simulink model "Plantv5"  (R2017a)
settings: Solver=FixedStepAuto  StartTime=0.0  StopTime=6000  FixedStep=.1  MaxStep=4.0  MinStep=.001  RelTol=1e-6
values from neighbouring files (symbols this model uses):
  B0 = 3.12e-5    (= 3.12e-05)    [starshot_DC_KD_setup.m]    (also in starshot_DC_setup.m; starshotmath.m; temp.m)
  G = 6.67e-11    [starshot_DC_KD_setup.m]    (also in starshot_DC_setup.m; temp.m)
  M_Earth = 5.972e24    (= 5.972e+24)    [starshot_DC_KD_setup.m]    (also in starshot_DC_setup.m; temp.m)
  q0 = [qmatlab(2:4),qmatlab(1)]'    [starshot_DC_KD_setup.m]    (also in starshot_DC_setup.m; temp.m)
  R_Earth = 6.378e6    (= 6378000)    [starshot_DC_KD_setup.m]    (also in starshot_DC_setup.m; temp.m)
undefined symbols (not defined in the file or in its folder): DiscIntNeverNeededParam, starshot
libraries: vrlib x2
settings Model: Creator=armen  LastModifiedBy=armen
settings OptimizationCC: DefaultParameterBehavior=Inlined  UseDivisionForNetSlopeComputation=on  UseFloatMulNetSlope=on  InlineInvariantSignals=on  PassReuseOutputArgsAs=Individual arguments  ZeroExternalMemoryAtStartup=off  ZeroInternalMemoryAtStartup=off  NoFixptDivByZeroProtection=on  EfficientFloat2IntCast=on  LifeSpan=1
settings DebuggingCC: ParameterTunabilityLossMsg=error  FrameProcessingCompatibilityMsg=none
settings HardwareCC: ProdBitPerPointer=32  ProdBitPerSizeT=32  ProdBitPerPtrDiffT=32  ProdLargestAtomicInteger=Long  ProdLargestAtomicFloat=Double  ProdWordSize=32  ProdHWDeviceType=ARM Compatible->ARM Cortex
settings SFSimCC: MATLABDynamicMemAlloc=off
settings RTWCC: SystemTargetFile=ert.tlc  TLCOptions=-aAlwaysIncludeCustomSrc=1  GenCodeOnly=on  TemplateMakefile=ert_default_tmf  Description=Embedded Coder  GenerateReport=on  IncludeHyperlinkInReport=on  LaunchReport=on  TargetLang=C++  GenerateTraceInfo=on  GenerateTraceReport=on  GenerateTraceReportSl=on  GenerateTraceReportSf=on  GenerateTraceReportEml=on
settings CodeAppCC: ForceParamTrailComments=on  IgnoreCustomStorageClasses=off  OperatorAnnotations=on  SimulinkDataObjDesc=on  SFDataObjDesc=on  MATLABFcnDesc=on  CustomSymbolStrGlobalVar=rt$N$M  CustomSymbolStrType=$N$M  CustomSymbolStrFcn=$N$M$F  CustomSymbolStrMacro=$N$M  InsertBlockDesc=on  MATLABSourceComments=on
settings ERTTargetCC: TargetLangStandard=C++03 (ISO)  GenerateSampleERTMain=on  IncludeMdlTerminateFcn=off  CombineSignalStateStructs=on  SupportAbsoluteTime=off  MultiInstanceERTCode=on  CodeInterfacePackaging=C++ class  SupportComplex=off  SupportNonInlinedSFcns=on  InlinedParameterPlacement=NonHierarchical  RootIOFormat=Structure reference  ERTCustomFileTemplate=example_file_process.tlc  ERTFilePackagingFormat=CompactWithDataFile

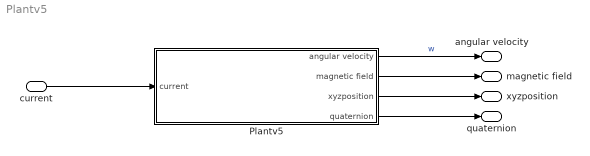
== system Plantv5 ==
  current : Inport  OutDataTypeStr=double  PortDimensions=3  SampleTime=[0.10000000000000001 0]  Interpolate=off
  Plantv5 : Subsystem  Tag=starshotsimv5  TreatAsAtomicUnit=on
      settings: RTWSystemCode=Inline
  angular velocity : Outport  OutDataTypeStr=double  PortDimensions=3  SampleTime=[0.10000000000000001 0]
  magnetic field : Outport  Port=2  OutDataTypeStr=double  PortDimensions=3  SampleTime=[0.10000000000000001 0]
  xyzposition : Outport  Port=3  OutDataTypeStr=double  PortDimensions=3  SampleTime=[0.10000000000000001 0]
  quaternion : Outport  Port=4  OutDataTypeStr=double  PortDimensions=4  SampleTime=[0.10000000000000001 0]
  wires:
  current/1 -> Plantv5/1(current)
  Plantv5/1(angular velocity) -> angular velocity/1  "w"
  Plantv5/2(magnetic field) -> magnetic field/1
  Plantv5/3(xyzposition) -> xyzposition/1
  Plantv5/4(quaternion) -> quaternion/1

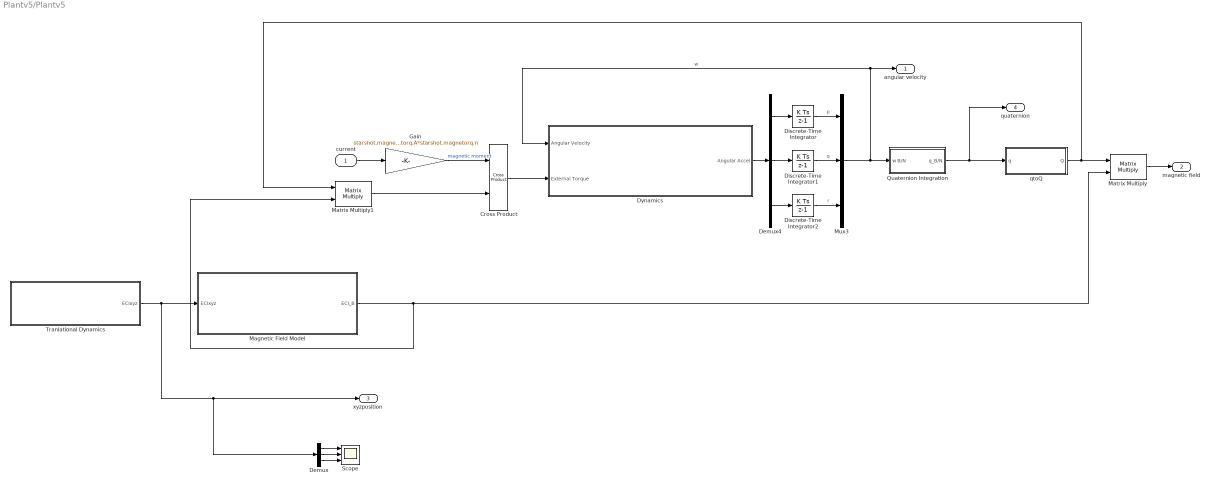
== system Plantv5/Plantv5 ==
  current : Inport
  Cross Product : vrlib/Utilities/Cross Product
      settings: SourceProductBaseCode=VR
  Demux : Demux  Outputs=3
  Demux4 : Demux  Outputs=3
  Discrete-Time Integrator : DiscreteIntegrator  InitialCondition=starshot.IC.w(1)  InitialConditionSetting=State (most efficient)  SampleTime=-1  ICPrevOutput=DiscIntNeverNeededParam  ICPrevScaledInput=DiscIntNeverNeededParam
  Discrete-Time Integrator1 : DiscreteIntegrator  InitialCondition=starshot.IC.w(2)  InitialConditionSetting=State (most efficient)  SampleTime=-1  ICPrevOutput=DiscIntNeverNeededParam  ICPrevScaledInput=DiscIntNeverNeededParam
  Discrete-Time Integrator2 : DiscreteIntegrator  InitialCondition=starshot.IC.w(3)  InitialConditionSetting=State (most efficient)  SampleTime=-1  ICPrevOutput=DiscIntNeverNeededParam  ICPrevScaledInput=DiscIntNeverNeededParam
  Dynamics : Subsystem  TreatAsAtomicUnit=on
  Gain : Gain  Gain=starshot.magnetorq.A*starshot.magnetorq.n
  Magnetic Field Model : Subsystem  TreatAsAtomicUnit=on
  Matrix Multiply : Product  Multiplication=Matrix(*)
  Matrix Multiply1 : Product  Multiplication=Matrix(*)
  Mux3 : Mux  Inputs=3
  Quaternion Integration : Subsystem
  Scope : Scope  NumInputPorts=3
  Tranlational Dynamics : Subsystem  TreatAsAtomicUnit=on
  qtoQ : Subsystem  TreatAsAtomicUnit=on
  angular velocity : Outport
  magnetic field : Outport  Port=2
  xyzposition : Outport  Port=3
  quaternion : Outport  Port=4
  wires:
  Matrix Multiply1/1 -> Cross Product/2
  qtoQ/1(Q) -> Matrix Multiply/1, Matrix Multiply1/1
  Demux/3 -> Scope/3
  Demux/1 -> Scope/1
  Demux/2 -> Scope/2
  Demux4/2 -> Discrete-Time Integrator1/1
  Discrete-Time Integrator/1 -> Mux3/1  "p"
  Cross Product/1 -> Dynamics/2(External Torque)
  Gain/1 -> Cross Product/1  "magnetic moment"
  current/1 -> Gain/1
  Mux3/1 -> angular velocity/1, Dynamics/1(Angular Velocity), Quaternion Integration/1(w B/N)  "w"
  Dynamics/1(Angular Accel) -> Demux4/1
  Quaternion Integration/1(q_B/N) -> qtoQ/1(q), quaternion/1
  Tranlational Dynamics/1(ECIxyz) -> Magnetic Field Model/1(ECIxyz), xyzposition/1, Demux/1
  Demux4/1 -> Discrete-Time Integrator/1
  Demux4/3 -> Discrete-Time Integrator2/1
  Discrete-Time Integrator2/1 -> Mux3/3  "r"
  Discrete-Time Integrator1/1 -> Mux3/2  "q"
  Magnetic Field Model/1(ECI_B) -> Matrix Multiply/2, Matrix Multiply1/2
  Matrix Multiply/1 -> magnetic field/1

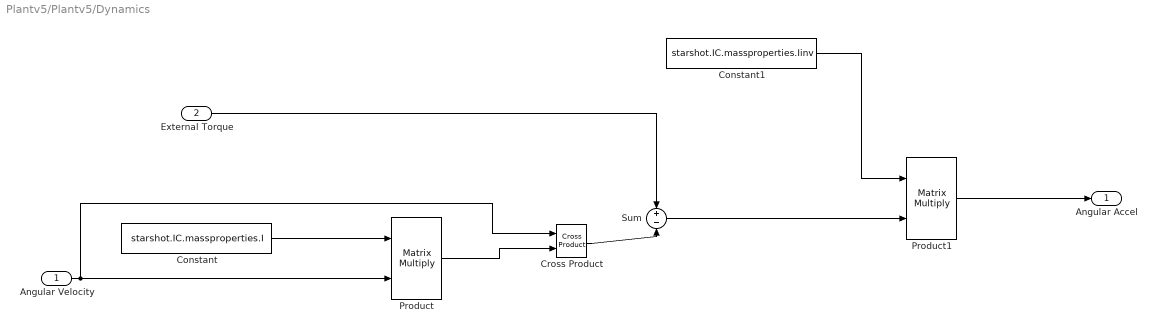
== system Plantv5/Plantv5/Dynamics ==
  Angular Velocity : Inport
  External Torque : Inport  Port=2
  Constant : Constant  Value=starshot.IC.massproperties.I
  Constant1 : Constant  Value=starshot.IC.massproperties.Iinv
  Cross Product : vrlib/Utilities/Cross Product
      settings: SourceProductBaseCode=VR
  Product : Product  Multiplication=Matrix(*)
  Product1 : Product  Multiplication=Matrix(*)
  Sum : Sum  Inputs=+-
  Angular Accel : Outport
  wires:
  Sum/1 -> Product1/2
  Product1/1 -> Angular Accel/1
  Constant1/1 -> Product1/1
  External Torque/1 -> Sum/1
  Product/1 -> Cross Product/2
  Cross Product/1 -> Sum/2
  Constant/1 -> Product/1
  Angular Velocity/1 -> Product/2, Cross Product/1

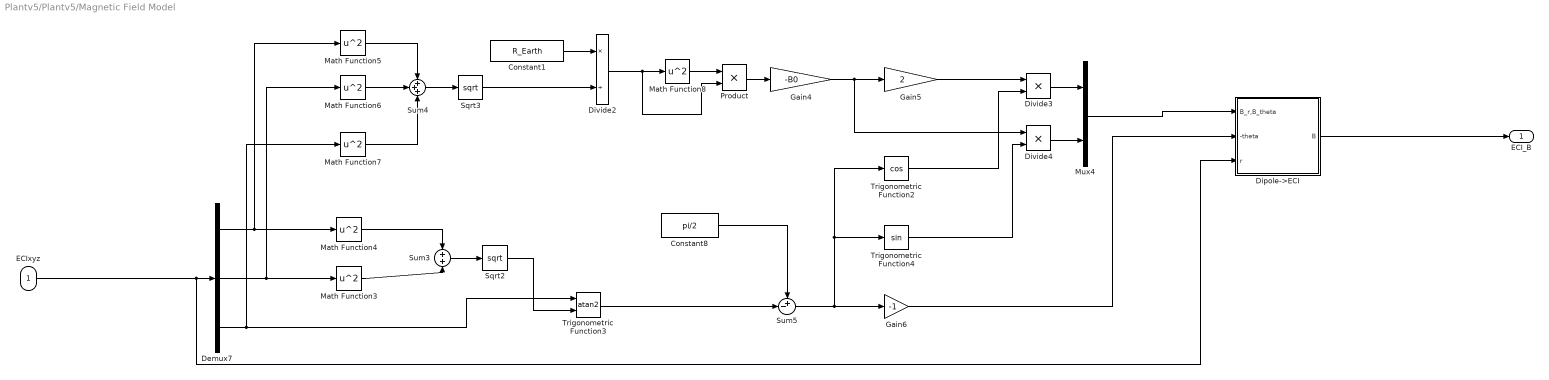
== system Plantv5/Plantv5/Magnetic Field Model ==
  ECIxyz : Inport
  Constant1 : Constant  Value=R_Earth
  Constant8 : Constant  Value=pi/2
  Demux7 : Demux  Outputs=3
  Dipole->ECI : Subsystem  TreatAsAtomicUnit=on
  Divide2 : Product  Inputs=*/
  Divide3 : Product  Inputs=**
  Divide4 : Product  Inputs=**
  Gain4 : Gain  Gain=-B0
  Gain5 : Gain  Gain=2
  Gain6 : Gain  Gain=-1
  Math Function{3..8} (6 alike) : Math  Operator=square  SaturateOnIntegerOverflow=on
  Mux4 : Mux  Inputs=2
  Product : Product
  Sqrt2 : Sqrt  SaturateOnIntegerOverflow=on
  Sqrt3 : Sqrt  SaturateOnIntegerOverflow=on
  Sum3 : Sum
  Sum4 : Sum  Inputs=+++
  Sum5 : Sum  Inputs=+-|
  Trigonometric Function2 : Trigonometry  Operator=cos
  Trigonometric Function3 : Trigonometry  Operator=atan2
  Trigonometric Function4 : Trigonometry
  ECI_B : Outport
  wires:
  ECIxyz/1 -> Demux7/1, Dipole->ECI/3(r)
  Divide3/1 -> Mux4/1
  Dipole->ECI/1(B) -> ECI_B/1
  Mux4/1 -> Dipole->ECI/1(B_r,B_theta)
  Constant8/1 -> Sum5/1
  Trigonometric Function3/1 -> Sum5/2
  Divide4/1 -> Mux4/2
  Gain6/1 -> Dipole->ECI/2(-theta)
  Trigonometric Function4/1 -> Divide4/2
  Sum5/1 -> Gain6/1, Trigonometric Function4/1, Trigonometric Function2/1
  Demux7/2 -> Math Function3/1, Math Function6/1
  Math Function6/1 -> Sum4/2
  Trigonometric Function2/1 -> Divide3/2
  Gain4/1 -> Divide4/1, Gain5/1
  Demux7/1 -> Math Function4/1, Math Function5/1
  Math Function3/1 -> Sum3/2
  Sum3/1 -> Sqrt2/1
  Divide2/1 -> Math Function8/1, Product/2
  Sum4/1 -> Sqrt3/1
  Sqrt3/1 -> Divide2/2
  Gain5/1 -> Divide3/1
  Math Function8/1 -> Product/1
  Product/1 -> Gain4/1
  Sqrt2/1 -> Trigonometric Function3/2
  Demux7/3 -> Trigonometric Function3/1, Math Function7/1
  Math Function4/1 -> Sum3/1
  Math Function5/1 -> Sum4/1
  Constant1/1 -> Divide2/1
  Math Function7/1 -> Sum4/3

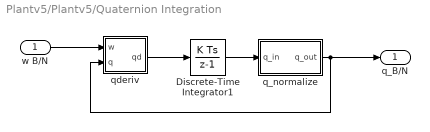
== system Plantv5/Plantv5/Quaternion Integration ==
  w B/N : Inport
  Discrete-Time Integrator1 : DiscreteIntegrator  InitialCondition=q0  InitialConditionSetting=State (most efficient)  SampleTime=-1  ICPrevOutput=DiscIntNeverNeededParam  ICPrevScaledInput=DiscIntNeverNeededParam
  q_normalize : Subsystem
  qderiv : Subsystem
  q_B/N : Outport
  wires:
  qderiv/1(qd) -> Discrete-Time Integrator1/1
  Discrete-Time Integrator1/1 -> q_normalize/1(q_in)
  q_normalize/1(q_out) -> q_B/N/1, qderiv/2(q)
  w B/N/1 -> qderiv/1(w)

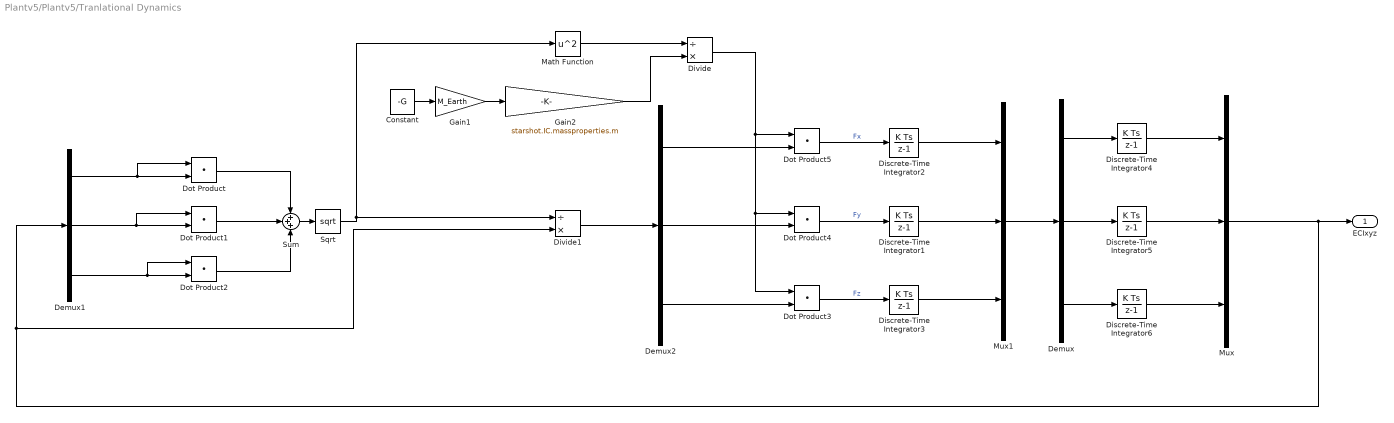
== system Plantv5/Plantv5/Tranlational Dynamics ==
  Constant : Constant  Value=-G
  Demux : Demux  Outputs=3
  Demux1 : Demux  Outputs=3
  Demux2 : Demux  Outputs=3
  Discrete-Time Integrator1 : DiscreteIntegrator  InitialCondition=starshot.IC.ydot  InitialConditionSetting=State (most efficient)  SampleTime=-1  ICPrevOutput=DiscIntNeverNeededParam  ICPrevScaledInput=DiscIntNeverNeededParam
  Discrete-Time Integrator2 : DiscreteIntegrator  InitialCondition=starshot.IC.xdot  InitialConditionSetting=State (most efficient)  SampleTime=-1  ICPrevOutput=DiscIntNeverNeededParam  ICPrevScaledInput=DiscIntNeverNeededParam
  Discrete-Time Integrator3 : DiscreteIntegrator  InitialCondition=starshot.IC.zdot  InitialConditionSetting=State (most efficient)  SampleTime=-1  ICPrevOutput=DiscIntNeverNeededParam  ICPrevScaledInput=DiscIntNeverNeededParam
  Discrete-Time Integrator4 : DiscreteIntegrator  InitialCondition=starshot.IC.x  InitialConditionSetting=State (most efficient)  SampleTime=-1  ICPrevOutput=DiscIntNeverNeededParam  ICPrevScaledInput=DiscIntNeverNeededParam
  Discrete-Time Integrator5 : DiscreteIntegrator  InitialCondition=starshot.IC.y  InitialConditionSetting=State (most efficient)  SampleTime=-1  ICPrevOutput=DiscIntNeverNeededParam  ICPrevScaledInput=DiscIntNeverNeededParam
  Discrete-Time Integrator6 : DiscreteIntegrator  InitialCondition=starshot.IC.z  InitialConditionSetting=State (most efficient)  SampleTime=-1  ICPrevOutput=DiscIntNeverNeededParam  ICPrevScaledInput=DiscIntNeverNeededParam
  Divide : Product  Inputs=/*
  Divide1 : Product  Inputs=/*
  Dot Product{,1..5} (6 alike) : DotProduct  InputSameDT=on  OutDataTypeStr=Inherit: Inherit via internal rule
  Gain1 : Gain  Gain=M_Earth
  Gain2 : Gain  Gain=starshot.IC.massproperties.m
  Math Function : Math  Operator=square  SaturateOnIntegerOverflow=on
  Mux : Mux  Inputs=3
  Mux1 : Mux  Inputs=3
  Sqrt : Sqrt  SaturateOnIntegerOverflow=on
  Sum : Sum  Inputs=+++
  ECIxyz : Outport
  wires:
  Mux/1 -> Demux1/1, Divide1/2, ECIxyz/1
  Discrete-Time Integrator2/1 -> Mux1/1
  Sqrt/1 -> Divide1/1, Math Function/1
  Gain2/1 -> Divide/2
  Divide1/1 -> Demux2/1
  Constant/1 -> Gain1/1
  Dot Product/1 -> Sum/1
  Dot Product5/1 -> Discrete-Time Integrator2/1  "Fx"
  Demux2/1 -> Dot Product5/2
  Gain1/1 -> Gain2/1
  Discrete-Time Integrator1/1 -> Mux1/2
  Math Function/1 -> Divide/1
  Demux2/3 -> Dot Product3/2
  Demux2/2 -> Dot Product4/2
  Dot Product2/1 -> Sum/3
  Demux1/3 -> Dot Product2/2, Dot Product2/1
  Dot Product1/1 -> Sum/2
  Divide/1 -> Dot Product5/1, Dot Product4/1, Dot Product3/1
  Dot Product3/1 -> Discrete-Time Integrator3/1  "Fz"
  Demux1/1 -> Dot Product/2, Dot Product/1
  Dot Product4/1 -> Discrete-Time Integrator1/1  "Fy"
  Sum/1 -> Sqrt/1
  Demux1/2 -> Dot Product1/2, Dot Product1/1
  Demux/2 -> Discrete-Time Integrator5/1
  Discrete-Time Integrator3/1 -> Mux1/3
  Mux1/1 -> Demux/1
  Demux/1 -> Discrete-Time Integrator4/1
  Demux/3 -> Discrete-Time Integrator6/1
  Discrete-Time Integrator4/1 -> Mux/1
  Discrete-Time Integrator5/1 -> Mux/2
  Discrete-Time Integrator6/1 -> Mux/3

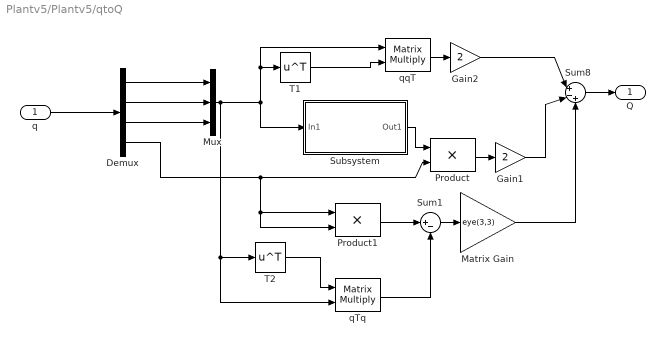
== system Plantv5/Plantv5/qtoQ ==
  q : Inport
  Demux : Demux
  Gain1 : Gain  Gain=2  SaturateOnIntegerOverflow=on  OutDataTypeStr=Inherit: Same as input  ParamDataTypeStr=Inherit: Same as input
  Gain2 : Gain  Gain=2  SaturateOnIntegerOverflow=on  OutDataTypeStr=Inherit: Same as input  ParamDataTypeStr=Inherit: Same as input
  Matrix Gain : Gain  Gain=eye(3,3)  SaturateOnIntegerOverflow=on  OutDataTypeStr=Inherit: Same as input  ParamDataTypeStr=Inherit: Same as input
  Mux : Mux  Inputs=3
  Product : Product  SaturateOnIntegerOverflow=on  InputSameDT=on  OutDataTypeStr=Inherit: Same as first input
  Product1 : Product  SaturateOnIntegerOverflow=on  InputSameDT=on  OutDataTypeStr=Inherit: Same as first input
  Subsystem : Subsystem
      mask Display: disp('3x3 cross matrix')
  Sum1 : Sum  Inputs=|+-  SaturateOnIntegerOverflow=on  InputSameDT=on  OutDataTypeStr=Inherit: Same as first input
  Sum8 : Sum  Inputs=|+-+  SaturateOnIntegerOverflow=on  InputSameDT=on  OutDataTypeStr=Inherit: Same as first input
  T1 : Math  Operator=transpose  SaturateOnIntegerOverflow=on
  T2 : Math  Operator=transpose  SaturateOnIntegerOverflow=on
  qTq : Product  Multiplication=Matrix(*)  SaturateOnIntegerOverflow=on  InputSameDT=on  OutDataTypeStr=Inherit: Same as first input
  qqT : Product  Multiplication=Matrix(*)  SaturateOnIntegerOverflow=on  InputSameDT=on  OutDataTypeStr=Inherit: Same as first input
  Q : Outport
  wires:
  Sum1/1 -> Matrix Gain/1
  qTq/1 -> Sum1/2
  Gain1/1 -> Sum8/2
  T1/1 -> qqT/2
  Gain2/1 -> Sum8/1
  Product1/1 -> Sum1/1
  Subsystem/1(Out1) -> Product/1
  Sum8/1 -> Q/1
  Mux/1 -> Subsystem/1(In1), T1/1, qqT/1, T2/1, qTq/2
  qqT/1 -> Gain2/1
  Product/1 -> Gain1/1
  Demux/4 -> Product/2, Product1/1, Product1/2
  T2/1 -> qTq/1
  Demux/3 -> Mux/3
  Demux/2 -> Mux/2
  Matrix Gain/1 -> Sum8/3
  Demux/1 -> Mux/1
  q/1 -> Demux/1

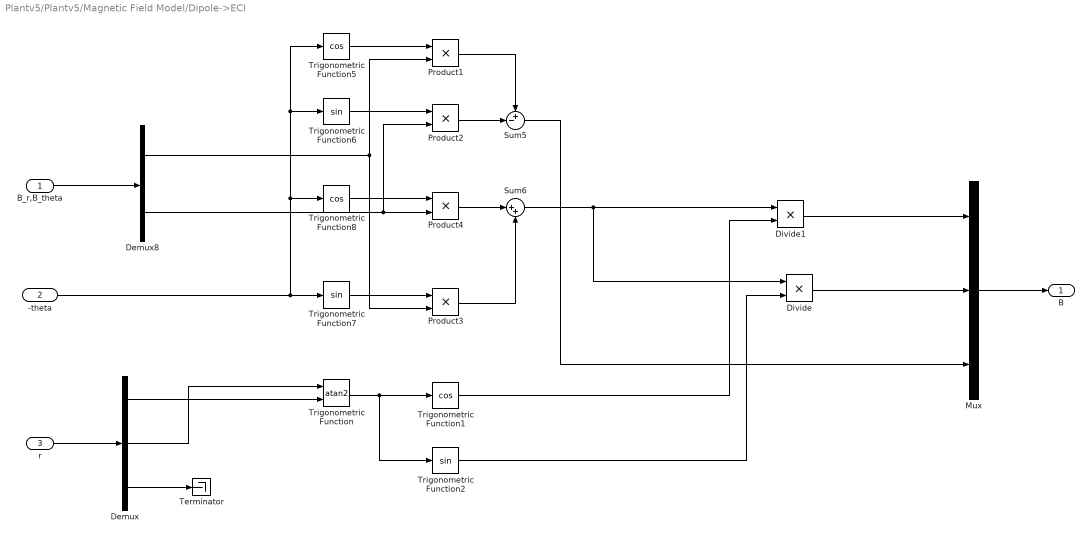
== system Plantv5/Plantv5/Magnetic Field Model/Dipole->ECI ==
  B_r,B_theta : Inport
  -theta : Inport  Port=2
  r : Inport  Port=3
  Demux : Demux  Outputs=3
  Demux8 : Demux  Outputs=2
  Divide : Product  Inputs=**
  Divide1 : Product  Inputs=**
  Mux : Mux  Inputs=3
  Product{1..4} (4 alike) : Product
  Sum5 : Sum  Inputs=+-|
  Sum6 : Sum  Inputs=|++
  Terminator : Terminator
  Trigonometric Function : Trigonometry  Operator=atan2
  Trigonometric Function1 : Trigonometry  Operator=cos
  Trigonometric Function2 : Trigonometry
  Trigonometric Function5 : Trigonometry  Operator=cos
  Trigonometric Function6 : Trigonometry
  Trigonometric Function7 : Trigonometry
  Trigonometric Function8 : Trigonometry  Operator=cos
  B : Outport
  wires:
  Divide/1 -> Mux/2
  Divide1/1 -> Mux/1
  Mux/1 -> B/1
  Trigonometric Function2/1 -> Divide/2
  Trigonometric Function1/1 -> Divide1/2
  Trigonometric Function/1 -> Trigonometric Function2/1, Trigonometric Function1/1
  Demux/1 -> Trigonometric Function/2
  Demux/2 -> Trigonometric Function/1
  Demux/3 -> Terminator/1
  r/1 -> Demux/1
  Product1/1 -> Sum5/1
  Sum6/1 -> Divide/1, Divide1/1
  Trigonometric Function6/1 -> Product2/1
  Trigonometric Function8/1 -> Product4/1
  Sum5/1 -> Mux/3
  B_r,B_theta/1 -> Demux8/1
  Trigonometric Function7/1 -> Product3/1
  Product2/1 -> Sum5/2
  Trigonometric Function5/1 -> Product1/1
  Demux8/2 -> Product4/2, Product2/2
  Demux8/1 -> Product1/2, Product3/2
  Product3/1 -> Sum6/2
  Product4/1 -> Sum6/1
  -theta/1 -> Trigonometric Function7/1, Trigonometric Function8/1, Trigonometric Function6/1, Trigonometric Function5/1

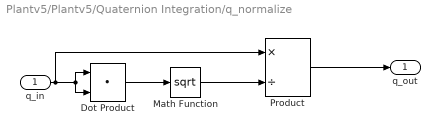
== system Plantv5/Plantv5/Quaternion Integration/q_normalize ==
  q_in : Inport  PortDimensions=4
  Dot Product : DotProduct  InputSameDT=on  OutDataTypeStr=Inherit: Inherit via internal rule
  Math Function : Math  Operator=sqrt  SaturateOnIntegerOverflow=on
  Product : Product  Inputs=*/  SaturateOnIntegerOverflow=on  InputSameDT=on  OutDataTypeStr=Inherit: Same as first input
  q_out : Outport
  wires:
  q_in/1 -> Product/1, Dot Product/1, Dot Product/2
  Dot Product/1 -> Math Function/1
  Math Function/1 -> Product/2
  Product/1 -> q_out/1

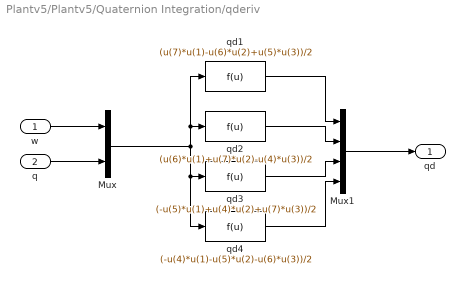
== system Plantv5/Plantv5/Quaternion Integration/qderiv ==
  w : Inport
  q : Inport  Port=2
  Mux : Mux  Inputs=2
  Mux1 : Mux
  qd1 : Fcn  Expr=(u(7)*u(1)-u(6)*u(2)+u(5)*u(3))/2
  qd2 : Fcn  Expr=(u(6)*u(1)+u(7)*u(2)-u(4)*u(3))/2
  qd3 : Fcn  Expr=(-u(5)*u(1)+u(4)*u(2)+u(7)*u(3))/2
  qd4 : Fcn  Expr=(-u(4)*u(1)-u(5)*u(2)-u(6)*u(3))/2
  qd : Outport
  wires:
  w/1 -> Mux/1
  q/1 -> Mux/2
  Mux/1 -> qd1/1, qd2/1, qd3/1, qd4/1
  qd1/1 -> Mux1/1
  qd2/1 -> Mux1/2
  qd3/1 -> Mux1/3
  qd4/1 -> Mux1/4
  Mux1/1 -> qd/1

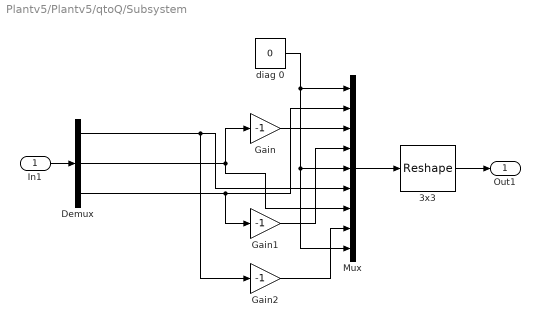
== system Plantv5/Plantv5/qtoQ/Subsystem ==
  In1 : Inport
  3x3 : Reshape  OutputDimensionality=Customize  OutputDimensions=[3,3]
  Demux : Demux  Outputs=3
  Gain : Gain  Gain=-1  SaturateOnIntegerOverflow=on  OutDataTypeStr=Inherit: Same as input  ParamDataTypeStr=Inherit: Same as input
  Gain1 : Gain  Gain=-1  SaturateOnIntegerOverflow=on  OutDataTypeStr=Inherit: Same as input  ParamDataTypeStr=Inherit: Same as input
  Gain2 : Gain  Gain=-1  SaturateOnIntegerOverflow=on  OutDataTypeStr=Inherit: Same as input  ParamDataTypeStr=Inherit: Same as input
  Mux : Mux  Inputs=9
  "diag 0 " : Constant  Value=0
  Out1 : Outport
  wires:
  In1/1 -> Demux/1
  3x3/1 -> Out1/1
  "diag 0 "/1 -> Mux/1, Mux/5, Mux/9
  Mux/1 -> 3x3/1
  Demux/3 -> Mux/2, Gain1/1
  Gain/1 -> Mux/3
  Demux/2 -> Gain/1, Mux/7
  Gain1/1 -> Mux/4
  Demux/1 -> Mux/6, Gain2/1
  Gain2/1 -> Mux/8
